simulink model "closedLoop_ProductionTest"  (R2022a)
settings: Solver=ode3  StartTime=0.0  StopTime=StopTime  FixedStep=Ts  RelTol=1e-3  EnableMultiTasking=on
values from neighbouring files (symbols this model uses):
  Aobs = [A-L*C]    [testClosedLoop_Design.m]    (also in testClosedLoop_Production.m)
  Bobs = [L, B-L*D]    [testClosedLoop_Design.m]    (also in testClosedLoop_Production.m)
  Cobs = eye(size(Aobs))    [testClosedLoop_Design.m]    (also in testClosedLoop_Production.m)
  Dobs = zeros(size(Bobs))    [testClosedLoop_Design.m]    (also in testClosedLoop_Production.m)
  Ts = 0.01    [conductOpenLoopTestonVirtualPlant.m]    (also in sineSweepOnVirtualPlant.m = 1/Fs)
undefined symbols (not defined in the file or in its folder): K
settings Model: Creator=Jon-L  LastModifiedBy=arifm
settings SolverCC: AlgebraicLoopSolver=TrustRegion
settings DataIOCC: SaveFormat=StructureWithTime  SignalLoggingSaveFormat=ModelDataLogs  SaveState=on  ReturnWorkspaceOutputs=off
settings OptimizationCC: ExpressionDepthLimit=2147483647  LifeSpan=inf
settings DebuggingCC: UnderspecifiedInitializationDetection=Classic  MergeDetectMultiDrivingBlocksExec=none  FcnCallInpInsideContextMsg=warning  UnconnectedInputMsg=warning  UnconnectedOutputMsg=warning  UnconnectedLineMsg=warning  AllowSymbolicDim=off  StateNameClashWarn=warning  SFUnexpectedBacktrackingDiag=warning  SFNoUnconditionalDefaultTransitionDiag=warning  SFExecutionAtInitializationDiag=none  SFMachineParentedDataDiag=warning  ArithmeticOperatorsInVariantConditions=warning
settings HardwareCC: ProdBitPerPointer=32  ProdBitPerSizeT=32  ProdBitPerPtrDiffT=32  ProdLargestAtomicFloat=None  ProdIntDivRoundTo=Undefined  ProdEndianess=Unspecified  ProdWordSize=32  ProdHWDeviceType=32-bit Generic
settings ModelReferenceCC: PropagateSignalLabelsOutOfModel=off
settings SFSimCC: SimUseLocalCustomCode=off  CustomCodeUndefinedFunction=UseInterfaceOnly
settings RTWCC: RTWUseLocalCustomCode=off  DLArmComputeVersion=19.05
settings CodeAppCC: StateflowObjectComments=on
settings GRTTargetCC: TargetLangStandard=C89/C90 (ANSI)  CombineOutputUpdateFcns=off  GRTInterface=on
settings ConfigComp: CovMetricSettings=dw  CovSaveCumulativeToWorkspaceVar=on  CovSaveSingleToWorkspaceVar=on  CovExternalEMLEnable=off

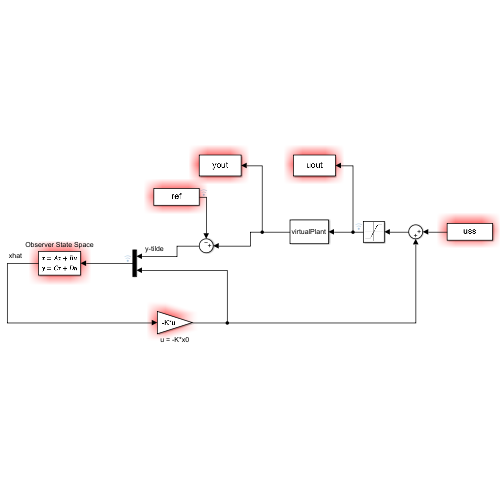
[thumbnail: Simulink's stored preview of the top-level diagram]
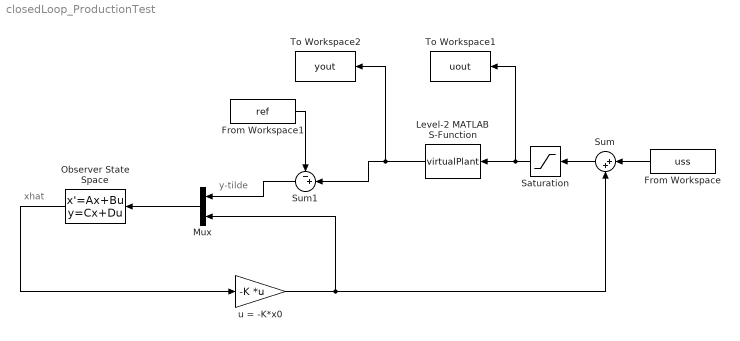
== system closedLoop_ProductionTest ==
  note: xhat
  note: y-tilde
  From Workspace : FromWorkspace  VariableName=uss
  From Workspace1 : FromWorkspace  VariableName=ref
  Level-2 MATLAB S-Function : M-S-Function  FunctionName=virtualPlant
  Mux : Mux  Inputs=2
  Observer State Space : StateSpace  A=Aobs  B=Bobs  C=Cobs  D=Dobs  InitialCondition=0  ParameterTunability=Unconstrained  ContinuousStateAttributes='observer_state'
  Saturation : Saturate  UpperLimit=10  LowerLimit=-10
  Sum : Sum  Inputs=|++
  Sum1 : Sum  Inputs=-+|
  To Workspace1 : ToWorkspace  VariableName=uout  SaveFormat=Structure With Time  SampleTime=Ts
  To Workspace2 : ToWorkspace  VariableName=yout  SaveFormat=Structure With Time  SampleTime=Ts
  u = -K*x0 : Gain  Gain=-K  Multiplication=Matrix(K*u)
  wires:
  Mux/1 -> Observer State Space/1
  Observer State Space/1 -> u = -K*x0/1
  Sum/1 -> Saturation/1
  u = -K*x0/1 -> Mux/2, Sum/2
  Level-2 MATLAB S-Function/1 -> To Workspace2/1, Sum1/2
  Sum1/1 -> Mux/1
  Saturation/1 -> Level-2 MATLAB S-Function/1, To Workspace1/1
  From Workspace/1 -> Sum/1
  From Workspace1/1 -> Sum1/1
